simulink model "forUTD5"  (R2022a)
settings: Solver=VariableStepAuto  StartTime=0.0  StopTime=100  RelTol=1e-3
settings Model: Creator=dtheilli  LastModifiedBy=julie
settings DebuggingCC: UnconnectedInputMsg=warning  UnconnectedOutputMsg=warning  UnconnectedLineMsg=warning
settings RTWCC: DLArmComputeVersion=19.05

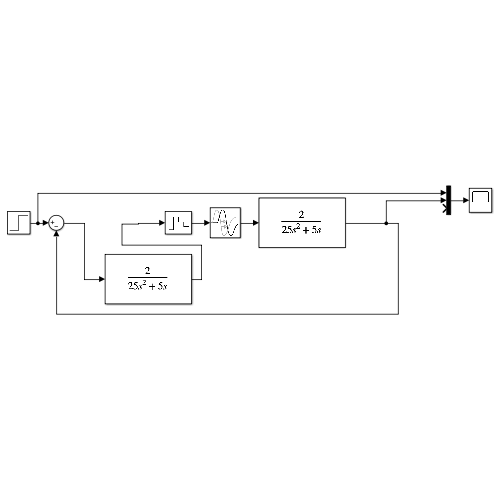
[thumbnail: Simulink's stored preview of the top-level diagram]
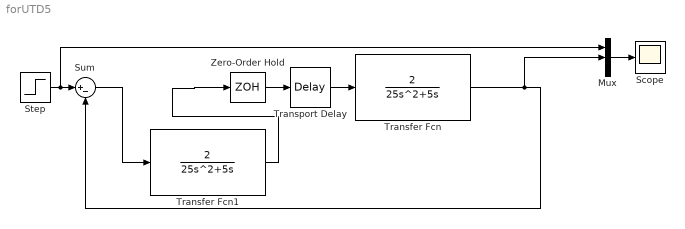
== system forUTD5 ==
  Mux : Mux  Inputs=3
  Scope : Scope
  Step : Step  Time=10  SampleTime=0
  Sum : Sum  Inputs=|+-
  Transfer Fcn : TransferFcn  Numerator=[2]  Denominator=[25 5 0]
  Transfer Fcn1 : TransferFcn  Numerator=[2]  Denominator=[25 5 0]
  Transport Delay : TransportDelay  DelayTime=2
  Zero-Order Hold : ZeroOrderHold  SampleTime=2
  wires:
  Transfer Fcn1/1 -> Zero-Order Hold/1
  Step/1 -> Mux/1, Sum/1
  Transfer Fcn/1 -> Mux/2, Sum/2
  Transport Delay/1 -> Transfer Fcn/1
  Zero-Order Hold/1 -> Transport Delay/1
  Mux/1 -> Scope/1
  Sum/1 -> Transfer Fcn1/1
